simulink model "fT"  (R2021a)
settings: Solver=VariableStepAuto  StartTime=0.0  StopTime=10  RelTol=1e-3
settings Model: Creator=luisd  LastModifiedBy=luisd

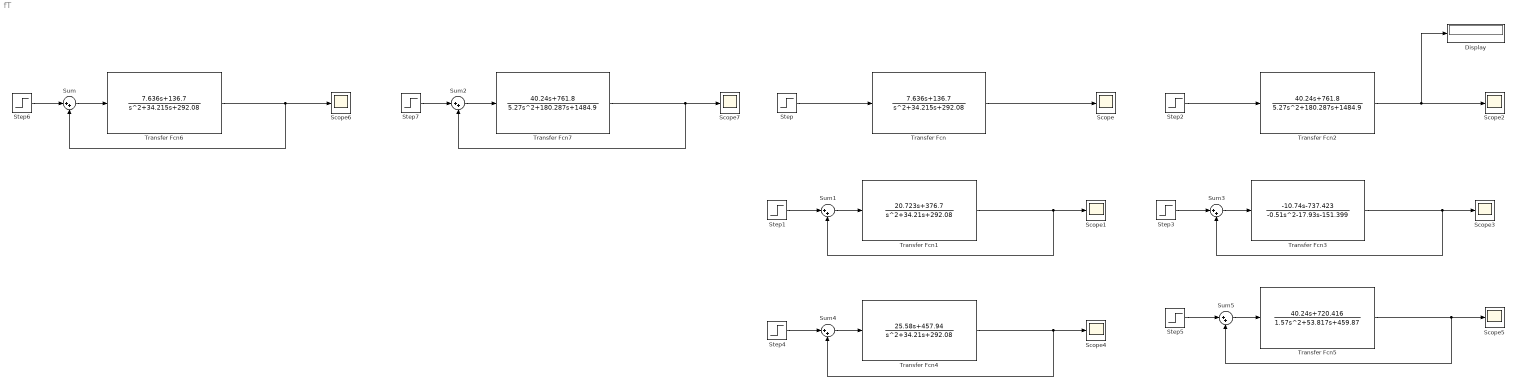
== system fT ==
  Display : Display
  Scope{,1..7} (8 alike) : Scope
  Step{,2,6..7} (4 alike) : Step  After=0.2  SampleTime=0
  Step{1,3..5} (4 alike) : Step  SampleTime=0
  Sum{,1..5} (6 alike) : Sum  Inputs=|++
  Transfer Fcn : TransferFcn  Numerator=[7.636 136.7]  Denominator=[1 34.215 292.08]
  Transfer Fcn1 : TransferFcn  Numerator=[20.723 376.7]  Denominator=[1 34.21 292.08]
  Transfer Fcn2 : TransferFcn  Numerator=[40.24 761.8]  Denominator=[5.27 180.287 1484.9]
  Transfer Fcn3 : TransferFcn  Numerator=[-10.74 -737.423]  Denominator=[-0.51 -17.93 -151.399]
  Transfer Fcn4 : TransferFcn  Numerator=[25.58 457.94]  Denominator=[1 34.21 292.08]
  Transfer Fcn5 : TransferFcn  Numerator=[40.24 720.416]  Denominator=[1.57 53.817 459.87]
  Transfer Fcn6 : TransferFcn  Numerator=[7.636 136.7]  Denominator=[1 34.215 292.08]
  Transfer Fcn7 : TransferFcn  Numerator=[40.24 761.8]  Denominator=[5.27 180.287 1484.9]
  wires:
  Transfer Fcn/1 -> Scope/1
  Step/1 -> Transfer Fcn/1
  Step1/1 -> Sum1/1
  Sum1/1 -> Transfer Fcn1/1
  Transfer Fcn1/1 -> Sum1/2, Scope1/1
  Step2/1 -> Transfer Fcn2/1
  Step3/1 -> Sum3/1
  Sum3/1 -> Transfer Fcn3/1
  Transfer Fcn3/1 -> Sum3/2, Scope3/1
  Step4/1 -> Sum4/1
  Transfer Fcn4/1 -> Sum4/2, Scope4/1
  Sum4/1 -> Transfer Fcn4/1
  Transfer Fcn5/1 -> Sum5/2, Scope5/1
  Sum5/1 -> Transfer Fcn5/1
  Step5/1 -> Sum5/1
  Transfer Fcn6/1 -> Sum/2, Scope6/1
  Transfer Fcn7/1 -> Sum2/2, Scope7/1
  Step6/1 -> Sum/1
  Sum/1 -> Transfer Fcn6/1
  Step7/1 -> Sum2/1
  Sum2/1 -> Transfer Fcn7/1
  Transfer Fcn2/1 -> Display/1, Scope2/1
